simulink model "gm_optimized_timing_multi_module_phase_shift_generator_built_in_counter"  (R2025b)
settings: Solver=FixedStepDiscrete  StartTime=0.0  StopTime=10e3  RelTol=1e-3
libraries: simulink x2, hdlmdlgenlib x1, simulink_need_slupdate x1, hdlsllib x1
settings Model: Creator=KoayXianCong  LastModifiedBy=KoayXianCong
settings OptimizationCC: BlockReduction=off  ConditionallyExecuteInputs=off  DefaultParameterBehavior=Inlined  InheritOutputTypeSmallerThanSingle=on
settings DebuggingCC: ArtificialAlgebraicLoopMsg=error  InheritedTsInSrcMsg=none  SingleTaskRateTransMsg=error
settings HardwareCC: ProdBitPerPointer=32.0  ProdBitPerSizeT=32.0  ProdBitPerPtrDiffT=32.0  ProdLargestAtomicFloat=None  ProdIntDivRoundTo=Undefined  ProdEndianess=Unspecified  ProdWordSize=32.0  ProdHWDeviceType=ASIC/FPGA->ASIC/FPGA  TargetBitPerPointer=64.0  TargetBitPerSizeT=64.0  TargetBitPerPtrDiffT=64.0  TargetLongLongMode=on  TargetIntDivRoundTo=Zero  TargetEndianess=LittleEndian  TargetWordSize=64.0  TargetHWDeviceType=Custom Processor->MATLAB Host Computer  ProdEqTarget=off

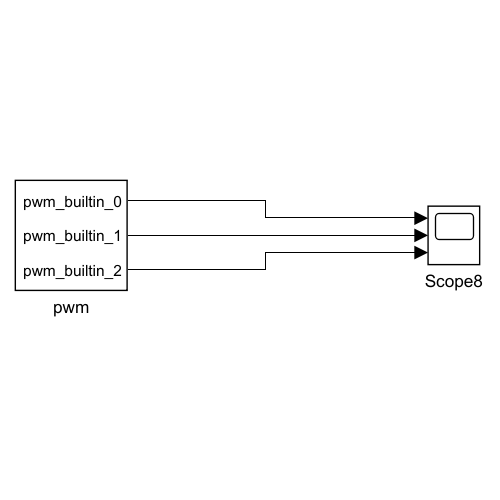
[thumbnail: Simulink's stored preview of the top-level diagram]
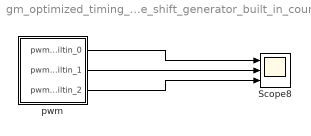
== system gm_optimized_timing_multi_module_phase_shift_generator_built_in_counter ==
  Scope8 : Scope  NumInputPorts=3
      settings: ActiveDisplayYMinimum=-1  ActiveDisplayYMaximum=1  DataLoggingVariableName=ScopeData10  DataLoggingSaveFormat=Array
  pwm : Subsystem
  wires:
  pwm/3(pwm_builtin_2) -> Scope8/3
  pwm/2(pwm_builtin_1) -> Scope8/2
  pwm/1(pwm_builtin_0) -> Scope8/1

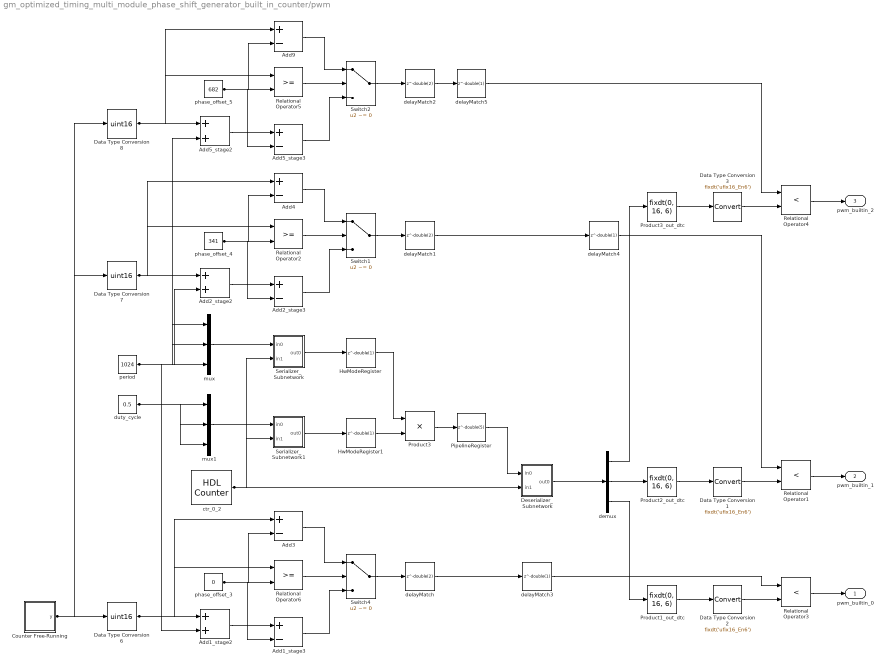
== system gm_optimized_timing_multi_module_phase_shift_generator_built_in_counter/pwm ==
  Add1_stage2 : Sum  OutDataTypeStr=fixdt(0, 17, 0)  AccumDataTypeStr=fixdt(1, 23, 4)  SampleTime=1
  Add1_stage3 : Sum  Inputs=+-  OutDataTypeStr=fixdt(1, 23, 4)  AccumDataTypeStr=fixdt(1, 23, 4)  SampleTime=1
  Add2_stage2 : Sum  OutDataTypeStr=fixdt(0, 17, 0)  AccumDataTypeStr=fixdt(1, 25, 7)  SampleTime=1
  Add2_stage3 : Sum  Inputs=+-  OutDataTypeStr=fixdt(1, 25, 7)  AccumDataTypeStr=fixdt(1, 25, 7)  SampleTime=1
  Add3 : Sum  Inputs=+-  OutDataTypeStr=fixdt(1, 22, 4)  AccumDataTypeStr=fixdt(1, 22, 4)  SampleTime=1
  Add4 : Sum  Inputs=+-  OutDataTypeStr=fixdt(1, 24, 7)  AccumDataTypeStr=fixdt(1, 24, 7)  SampleTime=1
  Add5_stage2 : Sum  OutDataTypeStr=fixdt(0, 17, 0)  AccumDataTypeStr=fixdt(1, 24, 6)  SampleTime=1
  Add5_stage3 : Sum  Inputs=+-  OutDataTypeStr=fixdt(1, 24, 6)  AccumDataTypeStr=fixdt(1, 24, 6)  SampleTime=1
  Add9 : Sum  Inputs=+-  OutDataTypeStr=fixdt(1, 23, 6)  AccumDataTypeStr=fixdt(1, 23, 6)  SampleTime=1
  Counter Free-Running : Subsystem  mask(Counter Free-Running){NumBits=double(10), tsamp=double(1)}
      mask prompts: NumBits "Simulink:masks:NumberOfBits_MP"; tsamp "Simulink:masks:SampleTime_MP"
      mask help: Simulink:masks:CounterFreeRunning_MD
  Data Type Conversion1 : DataTypeConversion  OutDataTypeStr=fixdt('ufix16_En6')
  Data Type Conversion2 : DataTypeConversion  OutDataTypeStr=fixdt('ufix16_En6')
  Data Type Conversion3 : DataTypeConversion  OutDataTypeStr=fixdt('ufix16_En6')
  Data Type Conversion6 : DataTypeConversion  OutDataTypeStr=uint16  SampleTime=1  SaturateOnIntegerOverflow=off  RndMeth=Floor
  Data Type Conversion7 : DataTypeConversion  OutDataTypeStr=uint16  SampleTime=1  SaturateOnIntegerOverflow=off  RndMeth=Floor
  Data Type Conversion8 : DataTypeConversion  OutDataTypeStr=uint16  SampleTime=1  SaturateOnIntegerOverflow=off  RndMeth=Floor
  Deserializer_Subnetwork : Subsystem
  HwModeRegister : Delay  DelayLength=double(1)  InitialCondition=0  SampleTime=0.333333333333333
  HwModeRegister1 : Delay  DelayLength=double(1)  InitialCondition=0  SampleTime=0.333333333333333
  PipelineRegister : Delay  DelayLength=double(5)  InitialCondition=0  SampleTime=0.333333333333333
  Product1_out_dtc : DataTypeConversion  OutDataTypeStr=fixdt(0, 16, 6)  SampleTime=1  SaturateOnIntegerOverflow=off  RndMeth=Floor
  Product2_out_dtc : DataTypeConversion  OutDataTypeStr=fixdt(0, 16, 6)  SampleTime=1  SaturateOnIntegerOverflow=off  RndMeth=Floor
  Product3 : Product  Inputs=**  OutDataTypeStr=fixdt(0, 32, 16)  SampleTime=0.333333333333333
  Product3_out_dtc : DataTypeConversion  OutDataTypeStr=fixdt(0, 16, 6)  SampleTime=1  SaturateOnIntegerOverflow=off  RndMeth=Floor
  Relational Operator1 : RelationalOperator  Operator=<  OutDataTypeStr=boolean  SampleTime=1  InputSameDT=off
  Relational Operator2 : RelationalOperator  OutDataTypeStr=boolean  SampleTime=1  InputSameDT=off
  Relational Operator3 : RelationalOperator  Operator=<  OutDataTypeStr=boolean  SampleTime=1  InputSameDT=off
  Relational Operator4 : RelationalOperator  Operator=<  OutDataTypeStr=boolean  SampleTime=1  InputSameDT=off
  Relational Operator5 : RelationalOperator  OutDataTypeStr=boolean  SampleTime=1  InputSameDT=off
  Relational Operator6 : RelationalOperator  OutDataTypeStr=boolean  SampleTime=1  InputSameDT=off
  Serializer_Subnetwork : Subsystem
  Serializer_Subnetwork1 : Subsystem
  Switch1 : Switch  Criteria=u2 ~= 0  Threshold="fi(0,0,1,0,\"hex\",\"0\")"  OutDataTypeStr=fixdt(1, 25, 7)  SampleTime=1  SaturateOnIntegerOverflow=off  InputSameDT=off
  Switch2 : Switch  Criteria=u2 ~= 0  Threshold="fi(0,0,1,0,\"hex\",\"0\")"  OutDataTypeStr=fixdt(1, 24, 6)  SampleTime=1  SaturateOnIntegerOverflow=off  InputSameDT=off
  Switch4 : Switch  Criteria=u2 ~= 0  Threshold="fi(0,0,1,0,\"hex\",\"0\")"  OutDataTypeStr=fixdt(1, 23, 4)  SampleTime=1  SaturateOnIntegerOverflow=off  InputSameDT=off
  ctr_0_2 : hdlsllib/Sources/HDL Counter  CountType=Count limited  CountInit=double(0)  CountStep=double(1)  CountMax=double(2)  CountFromType=Initial value  CountFrom=double(0)  CountResetPort=off  CountLoadPort=off  CountEnbPort=off  CountDirPort=off  CountHitOutputPort=off  CountDataType=Unsigned  CountWordLen=2  CountFracLen=0  CountSampTime=0.333333333333333
  delayMatch : Delay  DelayLength=double(2)  InitialCondition=0  SampleTime=1
  delayMatch1 : Delay  DelayLength=double(2)  InitialCondition=0  SampleTime=1
  delayMatch2 : Delay  DelayLength=double(2)  InitialCondition=0  SampleTime=1
  delayMatch3 : Delay  DelayLength=double(1)  InitialCondition=0  SampleTime=1
  delayMatch4 : Delay  DelayLength=double(1)  InitialCondition=0  SampleTime=1
  delayMatch5 : Delay  DelayLength=double(1)  InitialCondition=0  SampleTime=1
  demux : Demux  Outputs=3
  duty_cycle : Constant  Value=0.5  OutDataTypeStr=fixdt(0, 16, 16)  SampleTime=1
  mux : Mux  Inputs=3
  mux1 : Mux  Inputs=3
  period : Constant  Value=1024  OutDataTypeStr=uint16  SampleTime=1
  phase_offset_3 : Constant  Value=0  OutDataTypeStr=fixdt(1, 16, 4)  SampleTime=1
  phase_offset_4 : Constant  Value=341  OutDataTypeStr=fixdt(0, 16, 7)  SampleTime=1
  phase_offset_5 : Constant  Value=682  OutDataTypeStr=fixdt(0, 16, 6)  SampleTime=1
  pwm_builtin_0 : Outport  SampleTime=1
  pwm_builtin_1 : Outport  Port=2  SampleTime=1
  pwm_builtin_2 : Outport  Port=3  SampleTime=1
  wires:
  delayMatch1/1 -> delayMatch4/1
  Counter Free-Running/1(y) -> Data Type Conversion8/1, Data Type Conversion7/1, Data Type Conversion6/1
  Data Type Conversion8/1 -> Add9/1, Relational Operator5/1, Add5_stage2/1
  phase_offset_5/1 -> Add9/2, Relational Operator5/2, Add5_stage3/2
  period/1 -> mux/2, mux/1, mux/3, Add1_stage2/2, Add2_stage2/2, Add5_stage2/2
  Relational Operator3/1 -> pwm_builtin_0/1
  Add3/1 -> Switch4/1
  Data Type Conversion7/1 -> Add4/1, Relational Operator2/1, Add2_stage2/1
  demux/2 -> Product2_out_dtc/1
  Data Type Conversion6/1 -> Relational Operator6/1, Add3/1, Add1_stage2/1
  demux/1 -> Product3_out_dtc/1
  duty_cycle/1 -> mux1/3, mux1/2, mux1/1
  Add5_stage2/1 -> Add5_stage3/1
  phase_offset_4/1 -> Relational Operator2/2, Add2_stage3/2, Add4/2
  Add2_stage2/1 -> Add2_stage3/1
  Switch2/1 -> delayMatch2/1
  mux/1 -> Serializer_Subnetwork/1(in0)
  Product3_out_dtc/1 -> Data Type Conversion3/1
  mux1/1 -> Serializer_Subnetwork1/1(in0)
  Data Type Conversion1/1 -> Relational Operator1/2
  Add5_stage3/1 -> Switch2/3
  ctr_0_2/1 -> Deserializer_Subnetwork/2(in1), Serializer_Subnetwork1/2(in1), Serializer_Subnetwork/2(in1)
  phase_offset_3/1 -> Relational Operator6/2, Add3/2, Add1_stage3/2
  Switch1/1 -> delayMatch1/1
  Add1_stage2/1 -> Add1_stage3/1
  Relational Operator5/1 -> Switch2/2
  Add9/1 -> Switch2/1
  Add4/1 -> Switch1/1
  Relational Operator2/1 -> Switch1/2
  Relational Operator6/1 -> Switch4/2
  Add2_stage3/1 -> Switch1/3
  delayMatch3/1 -> Relational Operator3/1
  Serializer_Subnetwork/1(out0) -> HwModeRegister/1
  Serializer_Subnetwork1/1(out0) -> HwModeRegister1/1
  Add1_stage3/1 -> Switch4/3
  delayMatch/1 -> delayMatch3/1
  HwModeRegister/1 -> Product3/1
  HwModeRegister1/1 -> Product3/2
  Switch4/1 -> delayMatch/1
  Relational Operator4/1 -> pwm_builtin_2/1
  delayMatch2/1 -> delayMatch5/1
  Relational Operator1/1 -> pwm_builtin_1/1
  Product3/1 -> PipelineRegister/1
  delayMatch5/1 -> Relational Operator4/1
  PipelineRegister/1 -> Deserializer_Subnetwork/1(in0)
  Deserializer_Subnetwork/1(out0) -> demux/1
  delayMatch4/1 -> Relational Operator1/1
  demux/3 -> Product1_out_dtc/1
  Data Type Conversion2/1 -> Relational Operator3/2
  Product2_out_dtc/1 -> Data Type Conversion1/1
  Product1_out_dtc/1 -> Data Type Conversion2/1
  Data Type Conversion3/1 -> Relational Operator4/2

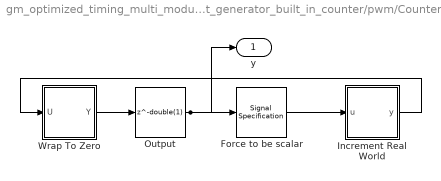
== system gm_optimized_timing_multi_module_phase_shift_generator_built_in_counter/pwm/Counter Free-Running ==
  Force to be scalar : SignalSpecification  OutDataTypeStr=fixdt(0, 10, 0)  Dimensions=1
  Increment Real World : Subsystem  mask(Real World Value Increment){}
      mask help: Simulink:masks:RealWorldValueIncrement_MD
      mask Display: disp('V++')
  Output : Delay  DelayLength=double(1)  InitialCondition=0  SampleTime=1
  Wrap To Zero : Subsystem  mask(Wrap To Zero){Threshold=double(1023)}
      mask prompts: Threshold "Simulink:masks:Threshold_MP"
      mask help: Simulink:masks:WrapToZero_MD
  y : Outport  SampleTime=1
  wires:
  Increment Real World/1(y) -> Wrap To Zero/1(U)
  Wrap To Zero/1(Y) -> Output/1
  Output/1 -> y/1, Force to be scalar/1
  Force to be scalar/1 -> Increment Real World/1(u)

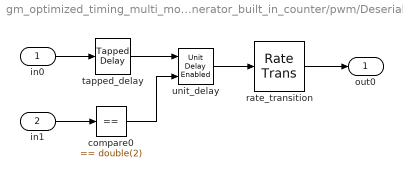
== system gm_optimized_timing_multi_module_phase_shift_generator_built_in_counter/pwm/Deserializer_Subnetwork ==
  in0 : Inport  OutDataTypeStr=fixdt(0, 32, 16)  SampleTime=0.333333333333333
  in1 : Inport  Port=2  OutDataTypeStr=fixdt(0, 2, 0)  SampleTime=0.333333333333333
  compare0 : simulink/Logic and Bit Operations/Compare To Constant  relop===  const=double(2)  OutDataTypeStr=boolean
  rate_transition : RateTransition  Integrity=off  Deterministic=off  OutPortSampleTimeOpt=Multiple of input port sample time  OutPortSampleTimeMultiple=3
  tapped_delay : simulink/Discrete/Tapped Delay  vinit=0  samptime=-1  NumDelays=double(2)  DelayOrder=Oldest  includeCurrent=on
  unit_delay : simulink_need_slupdate/Unit Delay Enabled  vinit=0.0  tsamp=-1
  out0 : Outport  OutDataTypeStr=fixdt(0, 32, 16)  PortDimensions=[3]  SampleTime=1
  wires:
  in0/1 -> tapped_delay/1
  unit_delay/1 -> rate_transition/1
  in1/1 -> compare0/1
  tapped_delay/1 -> unit_delay/1
  compare0/1 -> unit_delay/2
  rate_transition/1 -> out0/1

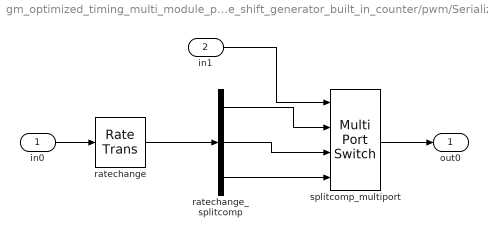
== system gm_optimized_timing_multi_module_phase_shift_generator_built_in_counter/pwm/Serializer_Subnetwork ==
  in0 : Inport  OutDataTypeStr=uint16  PortDimensions=[3]  SampleTime=1
  in1 : Inport  Port=2  OutDataTypeStr=fixdt(0, 2, 0)  SampleTime=0.333333333333333
  ratechange : RateTransition  Integrity=off  Deterministic=off  OutPortSampleTimeOpt=Multiple of input port sample time  OutPortSampleTimeMultiple=1/3
  ratechange_splitcomp : Demux  Outputs=3
  splitcomp_multiport : MultiPortSwitch  DataPortOrder=Zero-based contiguous  DiagnosticForDefault=None  zeroidx=on  OutDataTypeStr=uint16  SampleTime=0.333333333333333  SaturateOnIntegerOverflow=off  InputSameDT=off
  out0 : Outport  OutDataTypeStr=uint16  SampleTime=0.333333333333333
  wires:
  splitcomp_multiport/1 -> out0/1
  ratechange_splitcomp/1 -> splitcomp_multiport/2
  in0/1 -> ratechange/1
  ratechange/1 -> ratechange_splitcomp/1
  in1/1 -> splitcomp_multiport/1
  ratechange_splitcomp/3 -> splitcomp_multiport/4
  ratechange_splitcomp/2 -> splitcomp_multiport/3

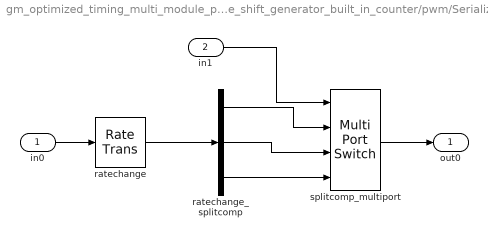
== system gm_optimized_timing_multi_module_phase_shift_generator_built_in_counter/pwm/Serializer_Subnetwork1 ==
  in0 : Inport  OutDataTypeStr=fixdt(0, 16, 16)  PortDimensions=[3]  SampleTime=1
  in1 : Inport  Port=2  OutDataTypeStr=fixdt(0, 2, 0)  SampleTime=0.333333333333333
  ratechange : RateTransition  Integrity=off  Deterministic=off  OutPortSampleTimeOpt=Multiple of input port sample time  OutPortSampleTimeMultiple=1/3
  ratechange_splitcomp : Demux  Outputs=3
  splitcomp_multiport : MultiPortSwitch  DataPortOrder=Zero-based contiguous  DiagnosticForDefault=None  zeroidx=on  OutDataTypeStr=fixdt(0, 16, 16)  SampleTime=0.333333333333333  SaturateOnIntegerOverflow=off  InputSameDT=off
  out0 : Outport  OutDataTypeStr=fixdt(0, 16, 16)  SampleTime=0.333333333333333
  wires:
  in0/1 -> ratechange/1
  ratechange/1 -> ratechange_splitcomp/1
  in1/1 -> splitcomp_multiport/1
  ratechange_splitcomp/1 -> splitcomp_multiport/2
  splitcomp_multiport/1 -> out0/1
  ratechange_splitcomp/2 -> splitcomp_multiport/3
  ratechange_splitcomp/3 -> splitcomp_multiport/4

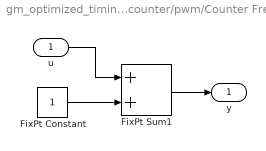
== system gm_optimized_timing_multi_module_phase_shift_generator_built_in_counter/pwm/Counter Free-Running/Increment Real World ==
  u : Inport  OutDataTypeStr=fixdt(0, 10, 0)  SampleTime=1
  FixPt Constant : Constant  OutDataTypeStr=fixdt(0, 10, 0)  SampleTime=1
  FixPt Sum1 : Sum  OutDataTypeStr=fixdt(0, 10, 0)  AccumDataTypeStr=fixdt(0, 11, 0)  SampleTime=1
  y : Outport  SampleTime=1
  wires:
  u/1 -> FixPt Sum1/1
  FixPt Constant/1 -> FixPt Sum1/2
  FixPt Sum1/1 -> y/1

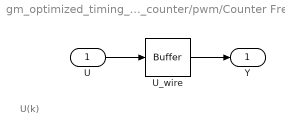
== system gm_optimized_timing_multi_module_phase_shift_generator_built_in_counter/pwm/Counter Free-Running/Wrap To Zero ==
  note: U(k)
  U : Inport  OutDataTypeStr=fixdt(0, 10, 0)  SampleTime=1
  U_wire : hdlmdlgenlib/Buffer
  Y : Outport  SampleTime=1  InitialOutput=0
  wires:
  U/1 -> U_wire/1
  U_wire/1 -> Y/1
